simulink model "EKF"  (R2025b)
settings: Solver=VariableStepAuto  StartTime=0.0  StopTime=60000  RelTol=1e-3
values from neighbouring files (symbols this model uses):
  AH = 2.5    [DataECM.sldd]
  C1_table = 14.038662996835537 14.038662996835537 14.038662996835537 14.038662996835537 14.038662996835537 14.038662996835537 14.038662996835537 14.038662996835537 14.038662996835537 13.716152424824331 13.70780042 13.70767275 15.4876125 15.52608855 15.37737691983936 15.37737691983936 15.37737691983936 15.37737691983936 15.37737691983936 15.37737691983936 15.37737691983936 14.359723373671073 14.359723373671073    [DataECM.sldd]
  C2_table = 1352.6468827825752 1352.6468827825752 1352.6468827825752 1352.6468827825752 1352.6468827825752 1352.6468827825752 1352.6468827825752 1352.6468827825752 1352.6468827825752 1358.3962866279012 1361.204699 1361.204668 1489.818558 1489.818563 1453.2108509645884 1453.2108509645884 1453.2108509645884 1453.2108509645884 1453.2108509645884 1453.2108509645884 1453.2108509645884 1344.0891535651501 1344.08915    [DataECM.sldd]
  Crate_bp = 0.25 0.5 1.0 2.0 5.0 8.0 10.0 15.0    [DataECM.sldd]
  dOCV_dSOC = 0.027781714285714541 0.01547542857142865 0.0058217142857142964 0.0033885714285713854 0.0032759999999999382 0.0022801428571428859 0.0012010000000000521 0.00044399999999999995 0.00097771428571427057 0.0016271428571428491 0.00076014285714287588 0.0027192380952381079 0.011066857142857068 0.013698285714285597    [DataECM.sldd]
  OCV_smooth = 3.0858971428571413 3.1553514285714277 3.2019628571428562 3.2135685714285707 3.23584857142857 3.2627085714285697 3.2814514285714278 3.2867285714285708 3.2903314285714278 3.3062828571428562 3.3228742857142848 3.33 3.3636628571428564 3.4321542857142844    [DataECM.sldd]
  R0_table = 0.0013697001953677269 0.0013697001953677269 0.0013697001953677269 0.0013697001953677269 0.0013697001953677269 0.0013697001953677269 0.0013697001953677269 0.0013697001953677269 0.0013697001953677269 0.00047575923642928091 0.0003277717761 0.0003277717761 0.0003841075501 0.0003841075501 0.00047396535261650448 0.00047396535261650448 0.00047396535261650448 0.00047396535261650448 0.00047396535261650448    [DataECM.sldd]
  R1_table = 0.0084007312474261228 0.0084007312474261228 0.0084007312474261228 0.0084007312474261228 0.0084007312474261228 0.0084007312474261228 0.0084007312474261228 0.0084007312474261228 0.0084007312474261228 0.0084955040256046478 0.008506708375 0.008525806321 0.009190588347 0.009184896157 0.009050179402327798 0.009050179402327798 0.009050179402327798 0.009050179402327798 0.009050179402327798 0.0090501794023    [DataECM.sldd]
  R2_table = 0.015106319088391846 0.015106319088391846 0.015106319088391846 0.015106319088391846 0.015106319088391846 0.015106319088391846 0.015106319088391846 0.015106319088391846 0.015106319088391846 0.014877593755183665 0.01478557796 0.01478557796 0.01454122871 0.01454122871 0.014670782061069287 0.014670782061069287 0.014670782061069287 0.014670782061069287 0.014670782061069287 0.014670782061069287 0.014670    [DataECM.sldd]
  SOC0 = 0.5    [DataECM.sldd]
  SOC_bp = 0.0 5.0 10.0 15.0 20.0 25.0 30.0 35.0 40.0 45.0 50.0 55.0 60.0 65.0 70.0 75.0 80.0 85.0 90.0 95.0 100.0    [DataECM.sldd]
  Ts = 1.0    [DataECM.sldd]
libraries: dspstat3 x2
settings Model: DataDictionary=DataECM.sldd  Creator=yashn  LastModifiedBy=yashn

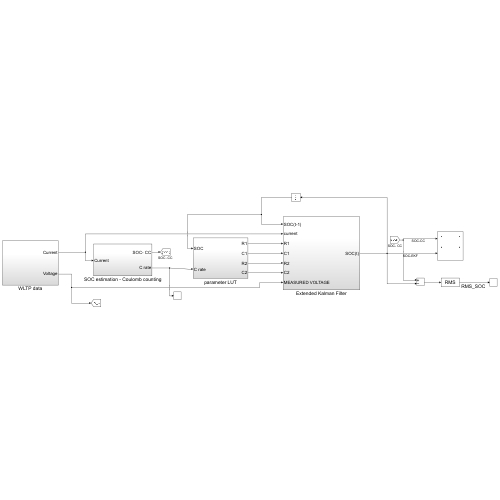
[thumbnail: Simulink's stored preview of the top-level diagram]
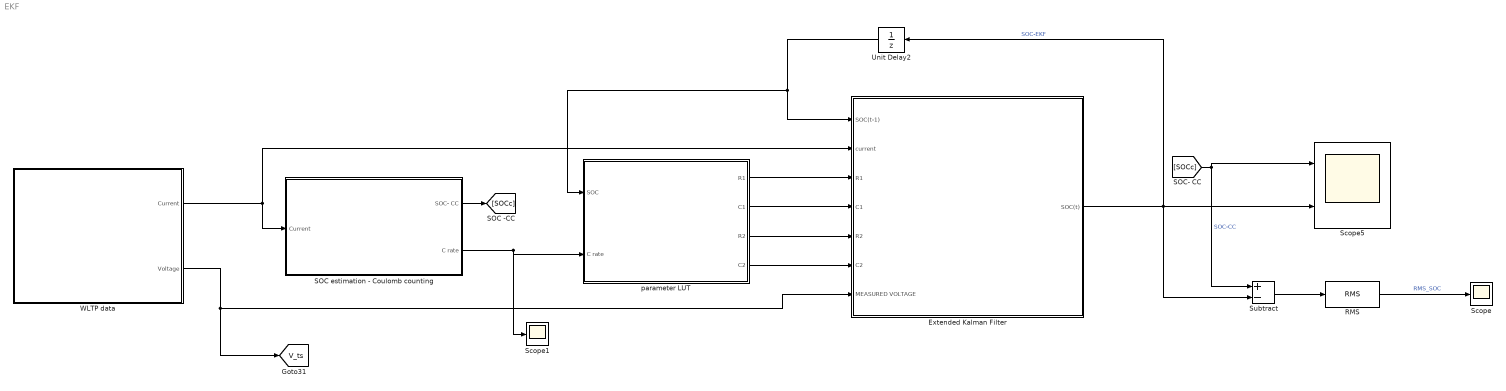
== system EKF ==
  Extended Kalman Filter : Subsystem
  RMS : dspstat3/RMS  run=off  directionMode=Each column  dimension=1  InputProcessing=Columns as channels (frame based)  reset_popup=None
  SOC estimation - Coulomb counting : Subsystem
  Scope : Scope
      settings: ActiveDisplayYMinimum=-5.907995751106168  ActiveDisplayYMaximum=53.174695797527647
  Scope1 : Scope
      settings: ActiveDisplayYMinimum=6.5789142605475206  ActiveDisplayYMaximum=24.732113284804708
  Scope5 : Scope  NumInputPorts=2
      settings: ActiveDisplayYMinimum=-6.7717206435124337  ActiveDisplayYMaximum=88.28121936496926  DataLoggingVariableName=ScopeData8
  Subtract : Sum  Inputs=+-
  Unit Delay2 : UnitDelay  SampleTime=-1  HasFrameUpgradeWarning=on
  WLTP data : Subsystem
  parameter LUT : Subsystem
  tag scope: V_ts=global
  wires:
  parameter LUT/3(R2) -> Extended Kalman Filter/5(R2)
  parameter LUT/1(R1) -> Extended Kalman Filter/3(R1)
  parameter LUT/2(C1) -> Extended Kalman Filter/4(C1)
  parameter LUT/4(C2) -> Extended Kalman Filter/6(C2)
  RMS/1 -> Scope/1  "RMS_SOC"
  Subtract/1 -> RMS/1
  Unit Delay2/1 -> parameter LUT/1(SOC), Extended Kalman Filter/1(SOC(t-1))
  SOC estimation - Coulomb counting/2(C rate) -> Scope1/1, parameter LUT/2(C rate)
  WLTP data/2(Voltage) -> Extended Kalman Filter/7(MEASURED VOLTAGE), [V_ts]
  SOC estimation - Coulomb counting/1(SOC- CC) -> [SOCc]
  Extended Kalman Filter/1(SOC(t)) -> Scope5/2, Subtract/2, Unit Delay2/1  "SOC-EKF"
  [SOCc] -> Subtract/1, Scope5/1  "SOC-CC"
  WLTP data/1(Current) -> Extended Kalman Filter/2(current), SOC estimation - Coulomb counting/1(Current)

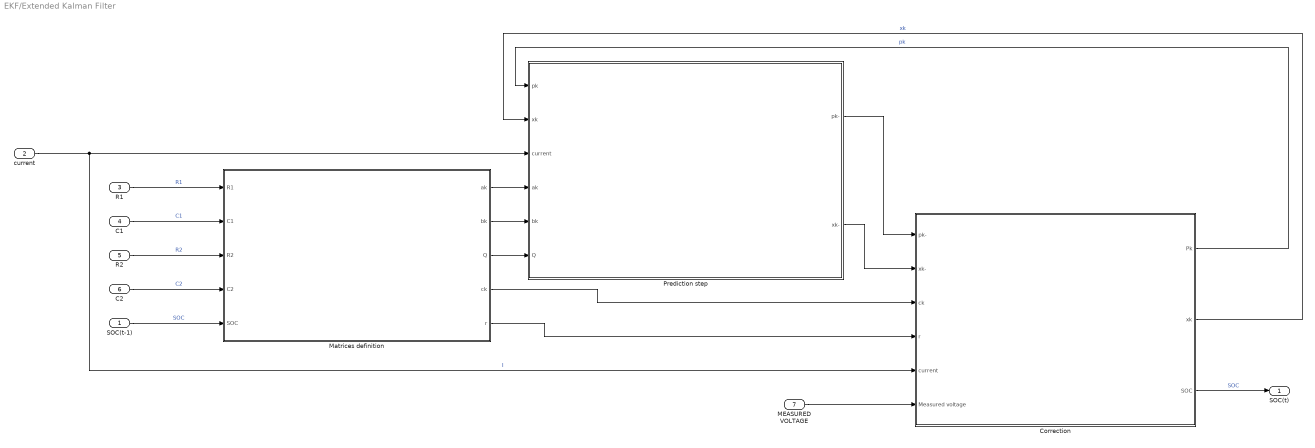
== system EKF/Extended Kalman Filter ==
  SOC(t-1) : Inport
  current : Inport  Port=2
  R1 : Inport  Port=3
  C1 : Inport  Port=4
  R2 : Inport  Port=5
  C2 : Inport  Port=6
  MEASURED VOLTAGE : Inport  Port=7
  Correction : Subsystem
  Matrices definition : Subsystem
  Prediction step : Subsystem
  SOC(t) : Outport
  wires:
  R1/1 -> Matrices definition/1(R1)  "R1"
  C1/1 -> Matrices definition/2(C1)  "C1"
  R2/1 -> Matrices definition/3(R2)  "R2"
  C2/1 -> Matrices definition/4(C2)  "C2"
  SOC(t-1)/1 -> Matrices definition/5(SOC)  "SOC"
  Prediction step/2(xk-) -> Correction/2(xk-)
  Correction/1(Pk) -> Prediction step/1(pk)  "pk"
  Matrices definition/3(Q) -> Prediction step/6(Q)
  Matrices definition/1(ak) -> Prediction step/4(ak)
  Matrices definition/2(bk) -> Prediction step/5(bk)
  Correction/2(xk) -> Prediction step/2(xk)  "xk"
  current/1 -> Correction/5(current), Prediction step/3(current)  "I"
  MEASURED VOLTAGE/1 -> Correction/6(Measured voltage)
  Prediction step/1(pk-) -> Correction/1(pk-)
  Matrices definition/4(ck) -> Correction/3(ck)
  Matrices definition/5(r) -> Correction/4(r)
  Correction/3(SOC) -> SOC(t)/1  "SOC"

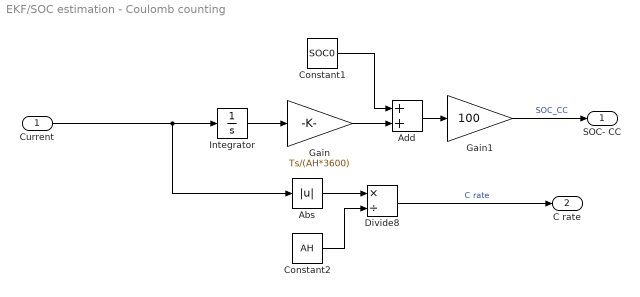
== system EKF/SOC estimation - Coulomb counting ==
  Current : Inport
  Abs : Abs  SaturateOnIntegerOverflow=off
  Add : Sum
  Constant1 : Constant  Value=SOC0
  Constant2 : Constant  Value=AH
  Divide8 : Product  Inputs=*/
  Gain : Gain  Gain=Ts/(AH*3600)
  Gain1 : Gain  Gain=100
  Integrator : Integrator
  SOC- CC : Outport
  C rate : Outport  Port=2
  wires:
  Integrator/1 -> Gain/1
  Gain1/1 -> SOC- CC/1  "SOC_CC"
  Constant2/1 -> Divide8/2
  Gain/1 -> Add/2
  Constant1/1 -> Add/1
  Abs/1 -> Divide8/1
  Add/1 -> Gain1/1
  Divide8/1 -> C rate/1  "C rate"
  Current/1 -> Abs/1, Integrator/1

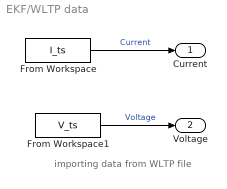
== system EKF/WLTP data ==
  note: importing data from WLTP file
  From Workspace : FromWorkspace  VariableName=I_ts  OutDataTypeStr=double  SampleTime=-1
  From Workspace1 : FromWorkspace  VariableName=V_ts  OutDataTypeStr=double  SampleTime=-1
  Current : Outport
  Voltage : Outport  Port=2
  wires:
  From Workspace/1 -> Current/1  "Current"
  From Workspace1/1 -> Voltage/1  "Voltage"

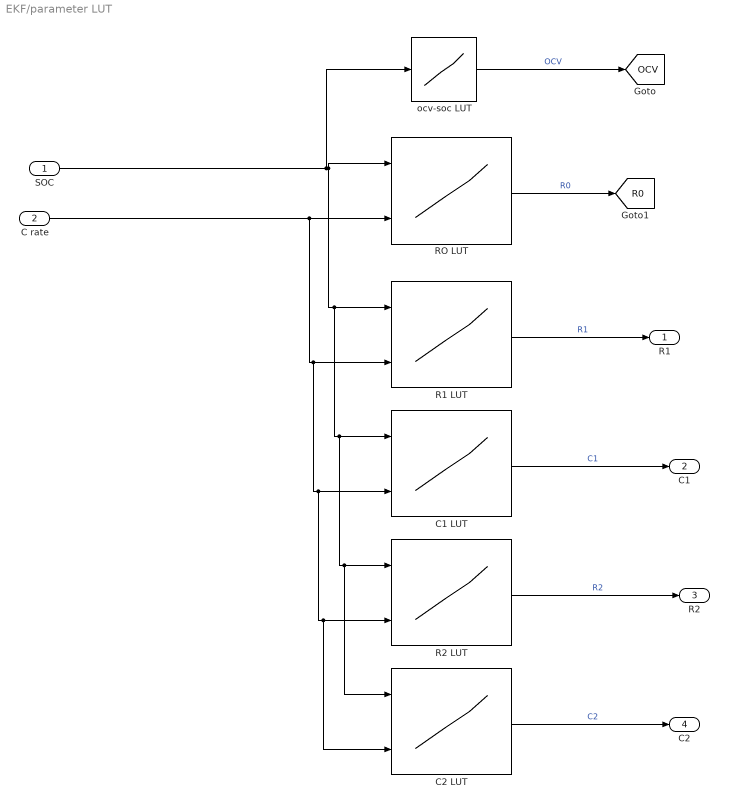
== system EKF/parameter LUT ==
  SOC : Inport
  C rate : Inport  Port=2
  C1 LUT : Lookup_n-D  BreakpointsForDimension1=SOC_bp  BreakpointsForDimension2=Crate_bp  BreakpointsForDimension3=[5, 7]  Table=C1_table  InterpMethod=Linear Lagrange  InternalRulePriority=Speed  RndMeth=Simplest
      settings: InputPortMap=u0,u1
  C2 LUT : Lookup_n-D  BreakpointsForDimension1=SOC_bp  BreakpointsForDimension2=Crate_bp  BreakpointsForDimension3=[5, 7]  Table=C2_table  InterpMethod=Linear Lagrange  InternalRulePriority=Speed  RndMeth=Simplest
      settings: InputPortMap=u0,u1
  R1 LUT : Lookup_n-D  BreakpointsForDimension1=SOC_bp  BreakpointsForDimension2=Crate_bp  BreakpointsForDimension3=[5, 7]  Table=R1_table  InterpMethod=Linear Lagrange  InternalRulePriority=Speed  RndMeth=Simplest
      settings: InputPortMap=u0,u1
  R2 LUT : Lookup_n-D  BreakpointsForDimension1=SOC_bp  BreakpointsForDimension2=Crate_bp  BreakpointsForDimension3=[5, 7]  Table=R2_table  InterpMethod=Linear Lagrange  InternalRulePriority=Speed  RndMeth=Simplest
      settings: InputPortMap=u0,u1
  RO LUT : Lookup_n-D  BreakpointsForDimension1=SOC_bp  BreakpointsForDimension2=Crate_bp  BreakpointsForDimension3=[5, 7]  Table=R0_table  InterpMethod=Linear Lagrange  InternalRulePriority=Speed  RndMeth=Simplest
      settings: InputPortMap=u0,u1
  ocv-soc LUT : Lookup_n-D  NumberOfTableDimensions=1  BreakpointsForDimension1=[2.5;5;10;15;20;30;40;50;60;70;80;90;95;100]  Table=[3.077;3.1749;3.1967;3.2132;3.2338;3.2636;3.2838;3.286;3.2892;3.3039;3.3274;3.3292;3.3316;3.4469]  InternalRulePriority=Speed  RndMeth=Simplest
  R1 : Outport
  C1 : Outport  Port=2
  R2 : Outport  Port=3
  C2 : Outport  Port=4
  tag scope: OCV=global, R0=global
  wires:
  R2 LUT/1 -> R2/1  "R2"
  C rate/1 -> C2 LUT/2, R2 LUT/2, C1 LUT/2, R1 LUT/2, RO LUT/2
  C2 LUT/1 -> C2/1  "C2"
  ocv-soc LUT/1 -> [OCV]  "OCV"
  C1 LUT/1 -> C1/1  "C1"
  SOC/1 -> ocv-soc LUT/1, C2 LUT/1, R2 LUT/1, C1 LUT/1, R1 LUT/1, RO LUT/1
  R1 LUT/1 -> R1/1  "R1"
  RO LUT/1 -> [R0]  "R0"

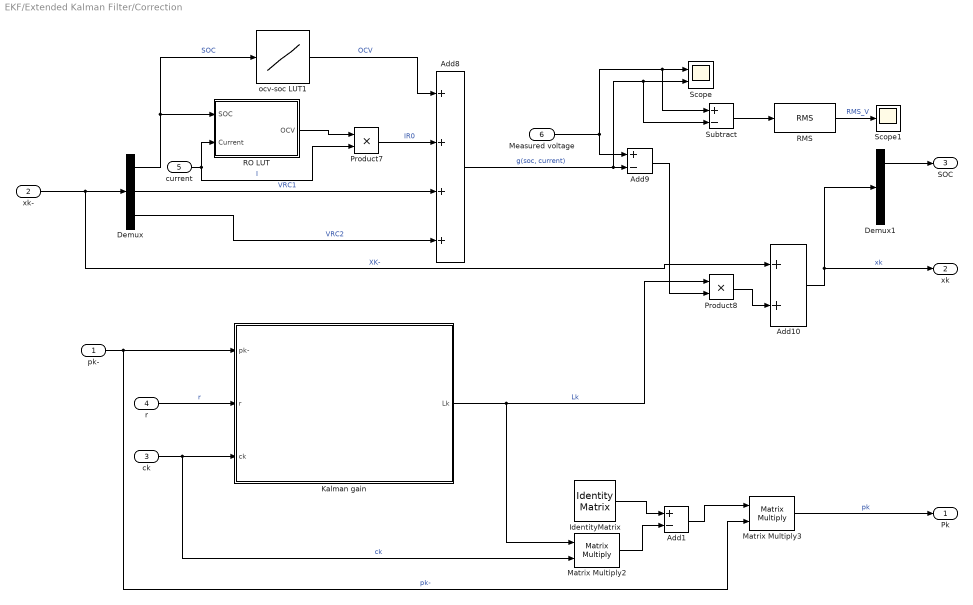
== system EKF/Extended Kalman Filter/Correction ==
  pk- : Inport
  xk- : Inport  Port=2
  ck : Inport  Port=3
  r : Inport  Port=4
  current : Inport  Port=5
  Measured voltage : Inport  Port=6
  Add1 : Sum  Inputs=+-
  Add10 : Sum
  Add8 : Sum  Inputs=++++
  Add9 : Sum  Inputs=+-
  Demux : Demux  Outputs=3
  Demux1 : Demux  Outputs=3
  IdentityMatrix : IdentityMatrix  OutputDimensions=3
  Kalman gain : Subsystem
  Matrix Multiply2 : Product  Multiplication=Matrix(*)
  Matrix Multiply3 : Product  Multiplication=Matrix(*)
  Product7 : Product
  Product8 : Product
  RMS : dspstat3/RMS  run=off  directionMode=Each column  dimension=1  InputProcessing=Columns as channels (frame based)  reset_popup=None
  RO LUT : Subsystem
  Scope : Scope  NumInputPorts=2
      settings: ActiveDisplayYMinimum=0.80373647473753618  ActiveDisplayYMaximum=5.2159824452908863  DataLoggingVariableName=ScopeData2
  Scope1 : Scope
      settings: ActiveDisplayYMinimum=-0.006753455587967248  ActiveDisplayYMaximum=0.060782048477501793  DataLoggingVariableName=ScopeData3
  Subtract : Sum  Inputs=+-
  ocv-soc LUT1 : Lookup_n-D  NumberOfTableDimensions=1  BreakpointsForDimension1=[2.5;5;10;15;20;30;40;50;60;70;80;90;95;100]  Table=[3.077;3.1749;3.1967;3.2132;3.2338;3.2636;3.2838;3.286;3.2892;3.3039;3.3274;3.3292;3.3316;3.4469]  InternalRulePriority=Speed  RndMeth=Simplest
  Pk : Outport
  xk : Outport  Port=2
  SOC : Outport  Port=3
  wires:
  Demux/1 -> ocv-soc LUT1/1, RO LUT/1(SOC)  "SOC"
  Product8/1 -> Add10/2
  Add8/1 -> Subtract/2, Scope/2, Add9/2  "g(soc, current)"
  Add10/1 -> xk/1, Demux1/1  "xk"
  current/1 -> RO LUT/2(Current), Product7/2  "I"
  Demux/3 -> Add8/4  "VRC2"
  Measured voltage/1 -> Add9/1, Subtract/1, Scope/1
  RO LUT/1(OCV) -> Product7/1
  Demux/2 -> Add8/3  "VRC1"
  Product7/1 -> Add8/2  "IR0"
  Kalman gain/1(Lk) -> Matrix Multiply2/1, Product8/1  "Lk"
  xk-/1 -> Add10/1, Demux/1  "XK-"
  Add9/1 -> Product8/2
  pk-/1 -> Matrix Multiply3/2, Kalman gain/1(pk-)  "pk-"
  Demux1/1 -> SOC/1
  r/1 -> Kalman gain/2(r)  "r"
  ck/1 -> Matrix Multiply2/2, Kalman gain/3(ck)  "ck"
  ocv-soc LUT1/1 -> Add8/1  "OCV"
  Matrix Multiply2/1 -> Add1/2
  IdentityMatrix/1 -> Add1/1
  Matrix Multiply3/1 -> Pk/1  "pk"
  Add1/1 -> Matrix Multiply3/1
  Subtract/1 -> RMS/1
  RMS/1 -> Scope1/1  "RMS_V"

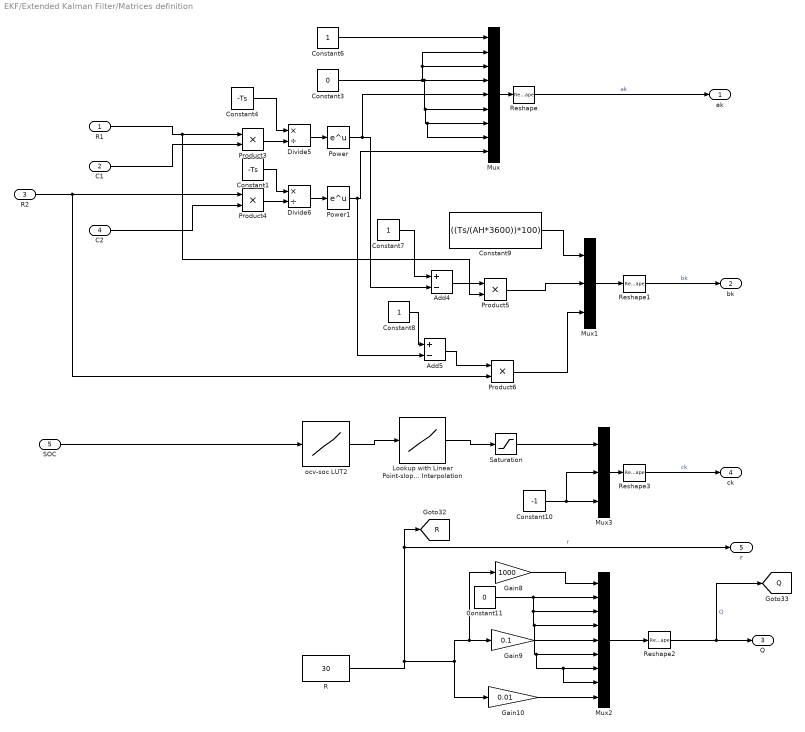
== system EKF/Extended Kalman Filter/Matrices definition ==
  R1 : Inport
  C1 : Inport  Port=2
  R2 : Inport  Port=3
  C2 : Inport  Port=4
  SOC : Inport  Port=5
  Add4 : Sum  Inputs=+-
  Add5 : Sum  Inputs=+-
  Constant1 : Constant  Value=-Ts
  Constant10 : Constant  Value=-1
  Constant11 : Constant  Value=0
  Constant3 : Constant  Value=0
  Constant4 : Constant  Value=-Ts
  Constant6 : Constant
  Constant7 : Constant
  Constant8 : Constant
  Constant9 : Constant  Value=((Ts/(AH*3600))*100)
  Divide5 : Product  Inputs=*/
  Divide6 : Product  Inputs=*/
  Gain10 : Gain  Gain=0.01
  Gain8 : Gain  Gain=1000
  Gain9 : Gain  Gain=0.1
  Lookup with Linear Point-slope Interpolation : Lookup_n-D  NumberOfTableDimensions=1  BreakpointsForDimension1=OCV_smooth  Table=dOCV_dSOC  InternalRulePriority=Speed  RndMeth=Simplest
  Mux : Mux  Inputs=9
  Mux1 : Mux  Inputs=3
  Mux2 : Mux  Inputs=9
  Mux3 : Mux  Inputs=3
  Power : Math
  Power1 : Math
  Product{3..6} (4 alike) : Product
  R : Constant  Value=30
  Reshape : Reshape  OutputDimensionality=Customize  OutputDimensions=[3,3]
  Reshape1 : Reshape  OutputDimensionality=Customize  OutputDimensions=[3,1]
  Reshape2 : Reshape  OutputDimensionality=Customize  OutputDimensions=[3,3]
  Reshape3 : Reshape  OutputDimensionality=Customize  OutputDimensions=[1,3]
  Saturation : Saturate  UpperLimit=0.7  LowerLimit=0.1
  ocv-soc LUT2 : Lookup_n-D  NumberOfTableDimensions=1  BreakpointsForDimension1=[2.5;5;10;15;20;30;40;50;60;70;80;90;95;100]  Table=[3.077;3.1749;3.1967;3.2132;3.2338;3.2636;3.2838;3.286;3.2892;3.3039;3.3274;3.3292;3.3316;3.4469]  InternalRulePriority=Speed  RndMeth=Simplest
  ak : Outport
  bk : Outport  Port=2
  Q : Outport  Port=3
  ck : Outport  Port=4
  r : Outport  Port=5
  tag scope: Q=global, R=global
  wires:
  Add4/1 -> Product5/1
  C1/1 -> Product3/2
  Divide5/1 -> Power/1
  Mux/1 -> Reshape/1
  Lookup with Linear Point-slope Interpolation/1 -> Saturation/1
  Constant9/1 -> Mux1/1
  Add5/1 -> Product6/1
  Reshape1/1 -> bk/1  "bk"
  Power1/1 -> Add5/2, Mux/9
  Constant6/1 -> Mux/1
  ocv-soc LUT2/1 -> Lookup with Linear Point-slope Interpolation/1
  Product5/1 -> Mux1/2
  Divide6/1 -> Power1/1
  Constant10/1 -> Mux3/3, Mux3/2
  Reshape3/1 -> ck/1  "ck"
  Constant3/1 -> Mux/2, Mux/3, Mux/8, Mux/7, Mux/6, Mux/4
  Constant4/1 -> Divide5/1
  Saturation/1 -> Mux3/1
  Product6/1 -> Mux1/3
  SOC/1 -> ocv-soc LUT2/1
  Power/1 -> Add4/2, Mux/5
  C2/1 -> Product4/2
  Product4/1 -> Divide6/2
  R2/1 -> Product4/1, Product6/2
  Constant8/1 -> Add5/1
  Product3/1 -> Divide5/2
  Mux3/1 -> Reshape3/1
  Constant7/1 -> Add4/1
  Reshape/1 -> ak/1  "ak"
  Mux1/1 -> Reshape1/1
  R1/1 -> Product5/2, Product3/1
  Constant1/1 -> Divide6/1
  Reshape2/1 -> Q/1, [Q]  "Q"
  R/1 -> Gain10/1, Gain9/1, Gain8/1, r/1, [R]  "r"
  Mux2/1 -> Reshape2/1
  Gain10/1 -> Mux2/9
  Gain8/1 -> Mux2/1
  Constant11/1 -> Mux2/8, Mux2/7, Mux2/6, Mux2/4, Mux2/3, Mux2/2
  Gain9/1 -> Mux2/5

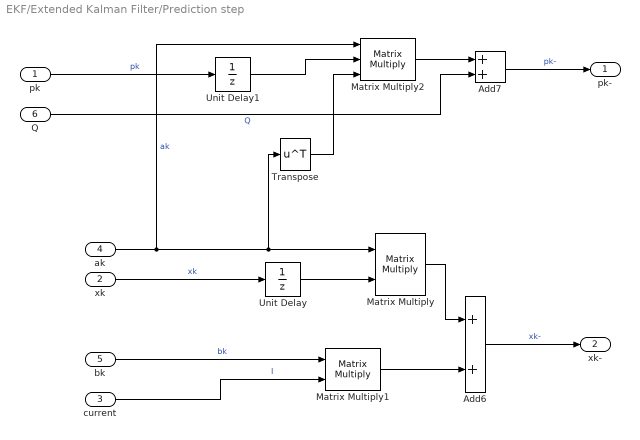
== system EKF/Extended Kalman Filter/Prediction step ==
  pk : Inport
  xk : Inport  Port=2
  current : Inport  Port=3
  ak : Inport  Port=4
  bk : Inport  Port=5
  Q : Inport  Port=6
  Add6 : Sum
  Add7 : Sum
  Matrix Multiply : Product  Multiplication=Matrix(*)
  Matrix Multiply1 : Product  Multiplication=Matrix(*)
  Matrix Multiply2 : Product  Inputs=3  Multiplication=Matrix(*)
  Transpose : Math  Operator=transpose
  Unit Delay : UnitDelay  SampleTime=-1  HasFrameUpgradeWarning=on
  Unit Delay1 : UnitDelay  SampleTime=-1  HasFrameUpgradeWarning=on
  pk- : Outport
  xk- : Outport  Port=2
  wires:
  Matrix Multiply2/1 -> Add7/1
  Matrix Multiply/1 -> Add6/1
  Unit Delay/1 -> Matrix Multiply/2
  ak/1 -> Matrix Multiply2/1, Transpose/1, Matrix Multiply/1  "ak"
  Q/1 -> Add7/2  "Q"
  Unit Delay1/1 -> Matrix Multiply2/2
  Matrix Multiply1/1 -> Add6/2
  Transpose/1 -> Matrix Multiply2/3
  Add7/1 -> pk-/1  "pk-"
  xk/1 -> Unit Delay/1  "xk"
  current/1 -> Matrix Multiply1/2  "I"
  bk/1 -> Matrix Multiply1/1  "bk"
  pk/1 -> Unit Delay1/1  "pk"
  Add6/1 -> xk-/1  "xk-"

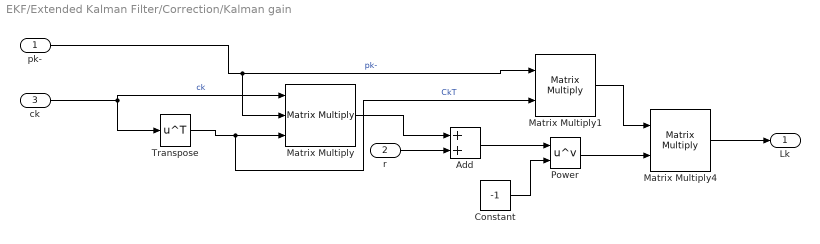
== system EKF/Extended Kalman Filter/Correction/Kalman gain ==
  pk- : Inport
  r : Inport  Port=2
  ck : Inport  Port=3
  Add : Sum
  Constant : Constant  Value=-1
  Matrix Multiply : Product  Inputs=3  Multiplication=Matrix(*)
  Matrix Multiply1 : Product  Multiplication=Matrix(*)
  Matrix Multiply4 : Product  Multiplication=Matrix(*)
  Power : Math  Operator=pow  SignedPower=on
  Transpose : Math  Operator=transpose
  Lk : Outport
  wires:
  Transpose/1 -> Matrix Multiply1/2, Matrix Multiply/3  "CkT"
  Matrix Multiply/1 -> Add/1
  r/1 -> Add/2
  Add/1 -> Power/1
  pk-/1 -> Matrix Multiply/2, Matrix Multiply1/1  "pk-"
  ck/1 -> Transpose/1, Matrix Multiply/1  "ck"
  Matrix Multiply4/1 -> Lk/1
  Matrix Multiply1/1 -> Matrix Multiply4/1
  Constant/1 -> Power/2
  Power/1 -> Matrix Multiply4/2

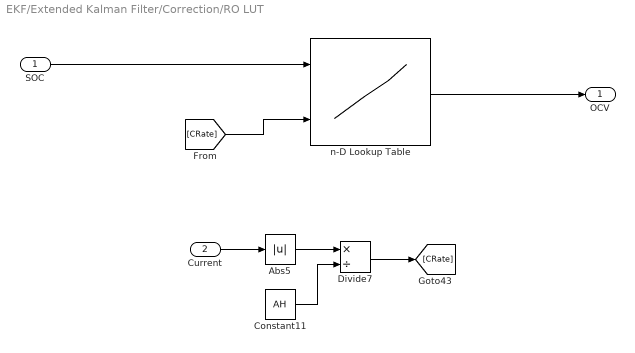
== system EKF/Extended Kalman Filter/Correction/RO LUT ==
  SOC : Inport
  Current : Inport  Port=2
  Abs5 : Abs  SaturateOnIntegerOverflow=off
  Constant11 : Constant  Value=AH
  Divide7 : Product  Inputs=*/
  n-D Lookup Table : Lookup_n-D  BreakpointsForDimension1=SOC_bp  BreakpointsForDimension2=Crate_bp  BreakpointsForDimension3=[5, 7]  Table=R0_table  InterpMethod=Linear Lagrange  InternalRulePriority=Speed  RndMeth=Simplest
      settings: InputPortMap=u0,u1
  OCV : Outport
  wires:
  Divide7/1 -> [CRate]
  Abs5/1 -> Divide7/1
  Current/1 -> Abs5/1
  Constant11/1 -> Divide7/2
  SOC/1 -> n-D Lookup Table/1
  [CRate] -> n-D Lookup Table/2
  n-D Lookup Table/1 -> OCV/1
